simulink model "VehicleModel"  (R2021b)
settings: Solver=ode4  StartTime=0.0  StopTime=150  FixedStep=0.0001  RelTol=1e-3
undefined symbols (not defined in the file): acc, gear, head, modelName, v0, x0, y0, yaw
settings Model: NumberOfSteps=1000  Creator=lenovo  LastModifiedBy=Lenovo

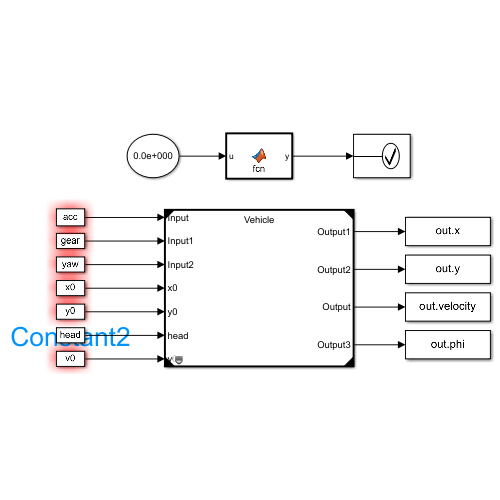
[thumbnail: Simulink's stored preview of the top-level diagram]
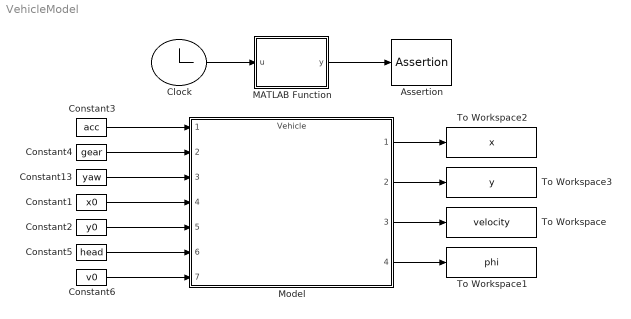
== system VehicleModel ==
  Assertion : Assertion  AssertionFailFcn=set_param(modelName,'SimulationCommand','pause')  StopWhenAssertionFail=off
  Clock : Clock
  Constant1 : Constant  Value=x0
  Constant13 : Constant  Value=yaw
  Constant2 : Constant  Value=y0
  Constant3 : Constant  Value=acc
  Constant4 : Constant  Value=gear
  Constant5 : Constant  Value=head
  Constant6 : Constant  Value=v0
  MATLAB Function : MATLAB Function  TreatAsAtomicUnit=on
  Model : ModelReference  ModelNameDialog=Vehicle.slxp  ModelReferenceVersion=5.15  CopyOfModelProtected=on
  To Workspace : ToWorkspace  VariableName=velocity  SaveFormat=Timeseries  SampleTime=-1
  To Workspace1 : ToWorkspace  VariableName=phi  SaveFormat=Timeseries  SampleTime=-1
  To Workspace2 : ToWorkspace  VariableName=x  SaveFormat=Timeseries  SampleTime=-1
  To Workspace3 : ToWorkspace  VariableName=y  SaveFormat=Timeseries  SampleTime=-1
  wires:
  Model/3 -> To Workspace/1
  Model/4 -> To Workspace1/1
  Model/2 -> To Workspace3/1
  Model/1 -> To Workspace2/1
  Constant3/1 -> Model/1
  Constant4/1 -> Model/2
  Constant13/1 -> Model/3
  Clock/1 -> MATLAB Function/1(u)
  MATLAB Function/1(y) -> Assertion/1
  Constant1/1 -> Model/4
  Constant2/1 -> Model/5
  Constant5/1 -> Model/6
  Constant6/1 -> Model/7

== matlab function VehicleModel/MATLAB Function ==
  data: u input; y output
function  y= fcn(u)
if u==0.1
    y=0;
else
    y=1;
end
